simulink model "constantvoltagek1"  (R2014a)
settings: Solver=ode45  StartTime=0.0  StopTime=10.0  RelTol=1e-3
libraries: powerlib x11, powerlib_extras x2, simulink_need_slupdate x1
settings Model: Creator=user  LastModifiedBy=CPGC
settings DebuggingCC: UnderspecifiedInitializationDetection=Classic  StateNameClashWarn=warning

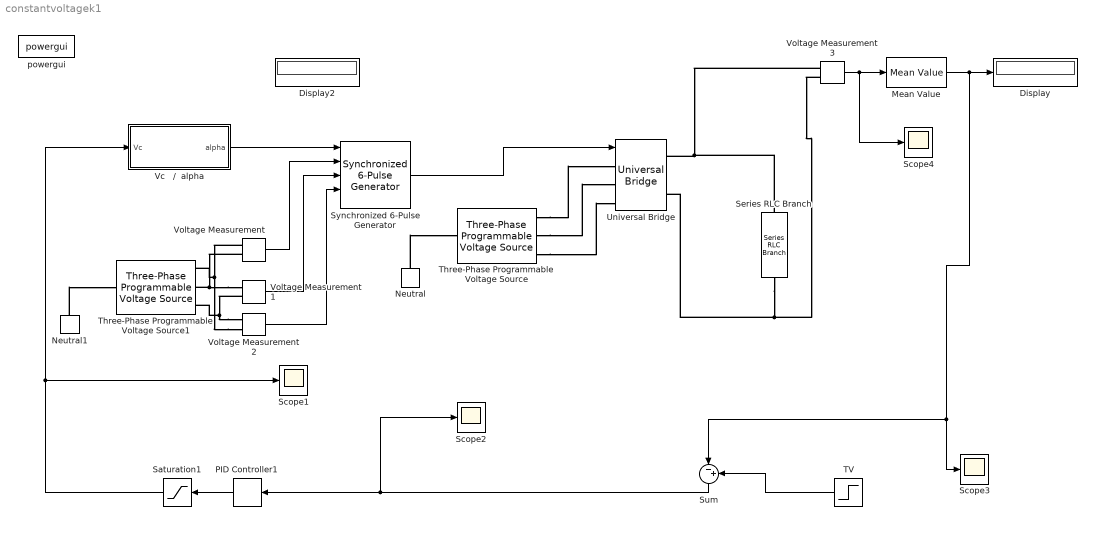
== system constantvoltagek1 ==
  Display : Display
  Display2 : Display
  Mean Value : powerlib_extras/Measurements/Mean Value  Period=1/50
  Neutral : powerlib/Elements/Neutral  LConnTagsString=a  NodeNumber=10
  Neutral1 : powerlib/Elements/Neutral  LConnTagsString=a  NodeNumber=10
  PID Controller1 : simulink_need_slupdate/PID Controller  P=2  I=20  D=0
  Saturation1 : Saturate  UpperLimit=3*1.414*230/pi  LowerLimit=-3*1.414*230/pi
  Scope{1..4} (4 alike) : Scope
      Scope1 settings: TimeRange=2  YMin=260  YMax=300
      Scope2 settings: TimeRange=2  YMin=0  YMax=16
      Scope3 settings: TimeRange=2  YMin=485  YMax=522.5  SaveName=ScopeData2
      Scope4 settings: TimeRange=2  YMin=-400  YMax=600  SaveName=ScopeData3
  Series RLC Branch : powerlib/Elements/Series RLC Branch  LConnTagsString=__new0  RConnTagsString=__new0  BranchType=RL  Resistance=10  Inductance=10  SetiL0=off  InitialCurrent=0  Capacitance=1e-6  Setx0=off  InitialVoltage=0  Measurements=None
  Sum : Sum  Inputs=|-+
  Synchronized 6-Pulse Generator : powerlib_extras/Control  Blocks/Synchronized 6-Pulse Generator  freq=50  pwidth=10  Double_Pulse=off
  TV : Step  Time=5  Before=500  After=200  SampleTime=0
  Three-Phase Programmable Voltage Source : powerlib/Electrical Sources/Three-Phase Programmable Voltage Source  PositiveSequence="[400  0 50]"  VariationEntity=None  VariationType=Step  VariationTypeAlt=Step  VariationStep=0.5  VariationRate=10  VariationMagnitude=0.3  VariationFrequency=2  VariationTiming=[1 2]  VariationPhaseA=off  Amplitudes=[1 0.8 1.2 1.0]  TimeValues=[0 0.1 0.15 0.2]  HarmonicGeneration=off  HarmonicA=[3 0.2 -25 0]  HarmonicB=[2 0.15 35 2]  Timing="[0.05  3]"  BusType=swing  Pref=0  Qref=0  Qmin=-inf  Qmax=inf
  Three-Phase Programmable Voltage Source1 : powerlib/Electrical Sources/Three-Phase Programmable Voltage Source  PositiveSequence="[1  0 50]"  VariationEntity=None  VariationType=Step  VariationTypeAlt=Step  VariationStep=0.5  VariationRate=10  VariationMagnitude=0.3  VariationFrequency=2  VariationTiming=[1 2]  VariationPhaseA=off  Amplitudes=[1 0.8 1.2 1.0]  TimeValues=[0 0.1 0.15 0.2]  HarmonicGeneration=off  HarmonicA=[3 0.2 -25 0]  HarmonicB=[2 0.15 35 2]  Timing="[0.05  3]"  BusType=swing  Pref=0  Qref=0  Qmin=-inf  Qmax=inf
  Universal Bridge : powerlib/Power Electronics/Universal Bridge  Arms=3  SnubberResistance=1e5  SnubberCapacitance=inf  Device=Thyristors  Ron=1e-3  Lon=0  ForwardVoltages="[  0  0  ]"  ForwardVoltage=0  GTOparameters=[ 10e-6 , 20e-6 ]  IGBTparameters=[ 1e-6 , 2e-6 ]  Measurements=None  Measurements_2=None  converterType=Rectifier
  "Vc   /  alpha " : Subsystem  TreatAsAtomicUnit=on
  Voltage Measurement{,1..3} (4 alike) : powerlib/Measurements/Voltage Measurement  PhasorSimulation=off  OutputType=Complex  PSBequivalent=0
  powergui : powerlib/powergui  SimulationMode=Discrete  SolverType=Tustin  SampleTime=50e-6  frequency=60  SPID=off  DisableSnubberDevices=off  DisableRonSwitches=off  DisableVfSwitches=off  SwTol=0  Interpol=off  DisplayEquations=off  Ts=0  methode=off  frequencyindice=50  Pbase=100e6  ErrMax=1e-4  Iterations=50  UnitsV=kV  UnitsW=MW  FunctionMessages=off  echomessages=off  HookPort=off  EnableUseOfTLC=off  x0status=blocks  RestoreLinks=warning  ResistiveCurrentMeasurement=off  Frange=[0:2:500]  Ylog=off  Xlog=on  ShowGrid=off  save=off  variable=ZData  structure=0  ZoomFFT=on  StartTime=0.0  cycles=1  DisplayStyle=1  fundamental=60  FreqAxis=off  MaxFrequency=1000  frequencyindicesteady=1  RmsSteady=1  display=off
  wires:
  Voltage Measurement/1 -> Synchronized 6-Pulse Generator/2
  Voltage Measurement1/1 -> Synchronized 6-Pulse Generator/3
  Voltage Measurement2/1 -> Synchronized 6-Pulse Generator/4
  Synchronized 6-Pulse Generator/1 -> Universal Bridge/1
  Voltage Measurement3/1 -> Scope4/1, Mean Value/1
  PID Controller1/1 -> Saturation1/1
  Mean Value/1 -> Sum/1, Scope3/1, Display/1
  Saturation1/1 -> Scope1/1, "Vc   /  alpha "/1(Vc)
  TV/1 -> Sum/2
  Sum/1 -> Scope2/1, PID Controller1/1
  "Vc   /  alpha "/1(alpha) -> Synchronized 6-Pulse Generator/1
  connections:
  Voltage Measurement1/LConn1 -- Three-Phase Programmable Voltage Source1/RConn2 -- Voltage Measurement/LConn2
  Voltage Measurement2/LConn2 -- Three-Phase Programmable Voltage Source1/RConn1 -- Voltage Measurement/LConn1
  Voltage Measurement2/LConn1 -- Three-Phase Programmable Voltage Source1/RConn3 -- Voltage Measurement1/LConn2
  Voltage Measurement3/LConn1 -- Series RLC Branch/LConn1 -- Universal Bridge/RConn1
  Voltage Measurement3/LConn2 -- Series RLC Branch/RConn1 -- Universal Bridge/RConn2
  Neutral/LConn1 -- Three-Phase Programmable Voltage Source/LConn1
  Neutral1/LConn1 -- Three-Phase Programmable Voltage Source1/LConn1
  Three-Phase Programmable Voltage Source/RConn1 -- Universal Bridge/LConn1
  Three-Phase Programmable Voltage Source/RConn2 -- Universal Bridge/LConn2
  Three-Phase Programmable Voltage Source/RConn3 -- Universal Bridge/LConn3

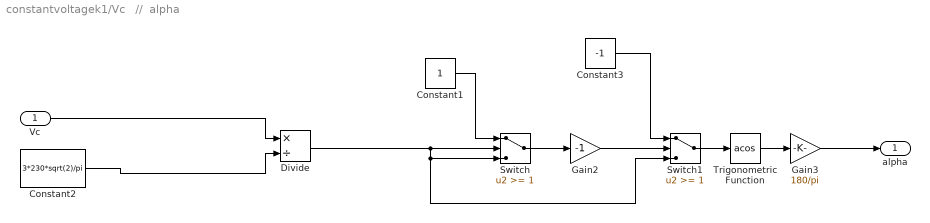
== system constantvoltagek1/Vc   //  alpha  ==
  Vc : Inport
  Constant1 : Constant
  Constant2 : Constant  Value=3*230*sqrt(2)/pi
  Constant3 : Constant  Value=-1
  Divide : Product  Inputs=*/
  Gain2 : Gain  Gain=-1
  Gain3 : Gain  Gain=180/pi
  Switch : Switch  Threshold=1
  Switch1 : Switch  Threshold=1
  Trigonometric Function : Trigonometry  Operator=acos
  alpha : Outport
  wires:
  Divide/1 -> Switch/2, Switch/3, Switch1/3
  Vc/1 -> Divide/1
  Constant2/1 -> Divide/2
  Constant1/1 -> Switch/1
  Constant3/1 -> Switch1/1
  Gain2/1 -> Switch1/2
  Switch/1 -> Gain2/1
  Switch1/1 -> Trigonometric Function/1
  Trigonometric Function/1 -> Gain3/1
  Gain3/1 -> alpha/1
